simulink model "problem8"  (R2020b)
settings: Solver=VariableStepAuto  StartTime=0.0  StopTime=10.0  RelTol=1e-3
settings Model: Creator=Varun  LastModifiedBy=Varun

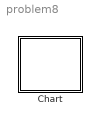
== system problem8 ==
  Chart : Stateflow chart  TreatAsAtomicUnit=on

== stateflow chart problem8/Chart ==
  state GroundFloor
    entry:
    status:
    during:
    currentFloor=0;
    checkFloor(currentFloor);
    exit:
    status=0;
  (default) -> GroundFloor
